simulink model "TransferBlockPT1"  (R2019b)
settings: Solver=ode45  StartTime=0.0  StopTime=10  MaxStep=0.02  RelTol=1e-3  EnableMultiTasking=on
model workspace (MAT data in the model file):
  AFS = 30
  AS = 0.5
settings Model: Creator=Reichl  LastModifiedBy=jakob
settings DataIOCC: SaveFormat=Array  ReturnWorkspaceOutputs=off  OutputSaveName=h
settings OptimizationCC: LifeSpan=inf
settings DebuggingCC: SolverPrmCheckMsg=warning  SFUnexpectedBacktrackingDiag=warning  SFNoUnconditionalDefaultTransitionDiag=warning  SFExecutionAtInitializationDiag=none  ArithmeticOperatorsInVariantConditions=warning
settings HardwareCC: ProdBitPerPointer=32  ProdBitPerSizeT=32  ProdBitPerPtrDiffT=32  ProdLargestAtomicFloat=None  ProdIntDivRoundTo=Undefined  ProdEndianess=Unspecified  ProdWordSize=32  ProdHWDeviceType=32-bit Generic
settings ModelReferenceCC: PropagateSignalLabelsOutOfModel=off
settings SFSimCC: SimUseLocalCustomCode=off  CustomCodeUndefinedFunction=UseInterfaceOnly
settings RTWCC: RTWUseLocalCustomCode=off
settings CodeAppCC: StateflowObjectComments=on
settings GRTTargetCC: TargetLangStandard=C89/C90 (ANSI)  GeneratePreprocessorConditionals=Disable all
settings ConfigComp: CovMetricSettings=dw  CovHtmlReporting=on  CovSaveCumulativeToWorkspaceVar=on  CovSaveSingleToWorkspaceVar=on  CovExternalEMLEnable=off  CovSFcnEnable=off

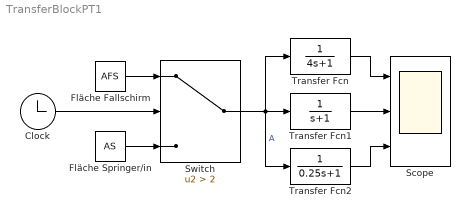
== system TransferBlockPT1 ==
  Clock : Clock
  Fläche Fallschirm : Constant  Value=AFS
  Fläche Springer/in : Constant  Value=AS
  Scope : Scope  NumInputPorts=3
  Switch : Switch  Criteria=u2 > Threshold  Threshold=2  ZeroCross=off
  Transfer Fcn : TransferFcn  Denominator=[4 1]
  Transfer Fcn1 : TransferFcn  Denominator=[1 1]
  Transfer Fcn2 : TransferFcn  Denominator=[0.25 1]
  wires:
  Clock/1 -> Switch/2
  Fläche Fallschirm/1 -> Switch/1
  Fläche Springer/in/1 -> Switch/3
  Switch/1 -> Transfer Fcn2/1, Transfer Fcn1/1, Transfer Fcn/1  "A"
  Transfer Fcn/1 -> Scope/1
  Transfer Fcn1/1 -> Scope/2
  Transfer Fcn2/1 -> Scope/3
